simulink model "statechart"  (R2015b)
settings: Solver=VariableStepAuto  StartTime=0.0  StopTime=10.0  RelTol=1e-3
settings Model: Creator=aleram  LastModifiedBy=Gabriel

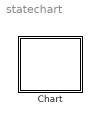
== system statechart ==
  Chart : Stateflow chart  TreatAsAtomicUnit=on

== stateflow chart statechart/Chart ==
  state Rotation
  state Line
  state Wait
  Line -> Rotation [order 2] : [event new goal]
  (default) -> Rotation : {x = 0
      | y = 0
      | theta = 0}
  Rotation -> Line : [abs(thetaR-theta) < 5 && abs(x0-x) < 2 && abs(y0-y) < 2]
  Wait -> Rotation : [Reset controller state]
  Line -> Wait [order 1] : [abs(xg-x) < 2 && abs(yg-y) < 2]
